simulink model "Joy"  (R2014a)
settings: Solver=ode3  StartTime=0.0  StopTime=inf  FixedStep=0.1  RelTol=1e-3
libraries: vrlib x1
settings Model: Creator=laca  LastModifiedBy=laca

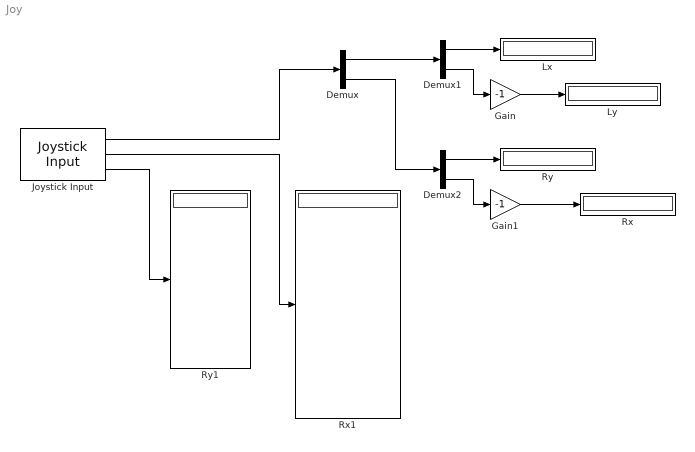
== system Joy ==
  Demux : Demux  Outputs=2
  Demux1 : Demux  Outputs=2
  Demux2 : Demux  Outputs=2
  Gain : Gain  Gain=-1
  Gain1 : Gain  Gain=-1
  Joystick Input : vrlib/Joystick Input  joyid=1  adjustports=on  forcefeed=off
  Lx : Display
  Ly : Display
  Rx : Display
  Rx1 : Display
  Ry : Display
  Ry1 : Display
  wires:
  Joystick Input/1 -> Demux/1
  Joystick Input/3 -> Ry1/1
  Demux/1 -> Demux1/1
  Demux1/1 -> Lx/1
  Demux1/2 -> Gain/1
  Demux/2 -> Demux2/1
  Demux2/1 -> Ry/1
  Demux2/2 -> Gain1/1
  Gain/1 -> Ly/1
  Gain1/1 -> Rx/1
  Joystick Input/2 -> Rx1/1
